simulink model "adaptiverror1 (1)"  (R2025a)
settings: Solver=VariableStepAuto  StartTime=0.0  StopTime=10.0  RelTol=1e-3
undefined symbols (not defined in the file): C1_LUT, C2_LUT, Current_table, OCV_table, R0_LUT, R1_LUT, R2_LUT, SOC_bp, SOC_bp_current, SOC_bp_ocv, Temp_bp
libraries: nesl_utility x13, fl_lib x11, ee_lib x2
settings Model: Creator=nandh  LastModifiedBy=nandh

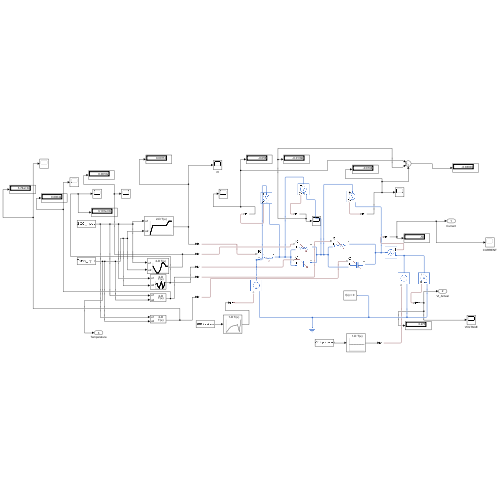
[thumbnail: Simulink's stored preview of the top-level diagram]
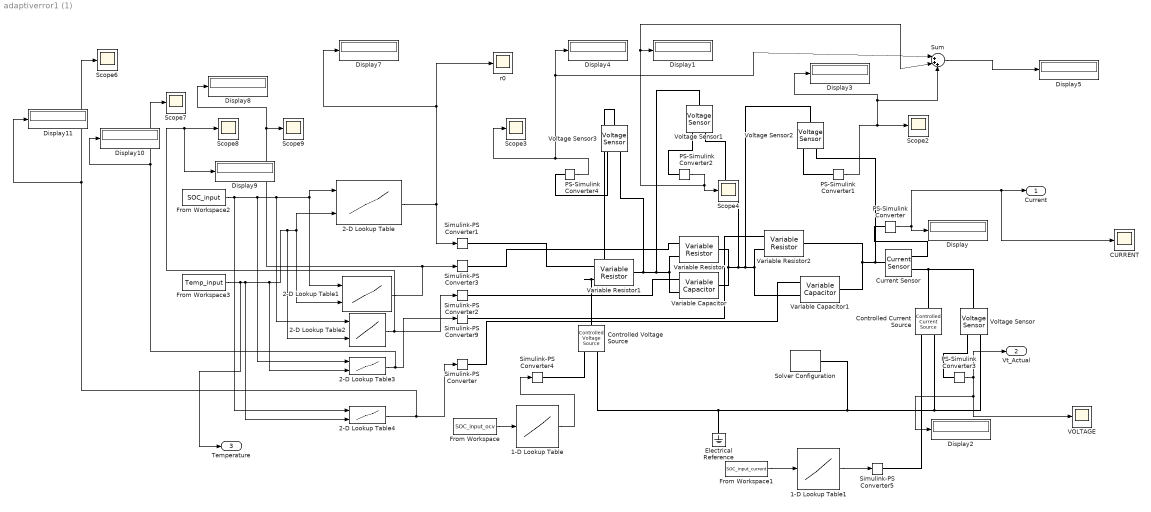
== system adaptiverror1 (1) ==
  1-D Lookup Table : Lookup_n-D  NumberOfTableDimensions=1  BreakpointsForDimension1=SOC_bp_ocv  Table=OCV_table  InternalRulePriority=Speed  RndMeth=Simplest
  1-D Lookup Table1 : Lookup_n-D  NumberOfTableDimensions=1  BreakpointsForDimension1=SOC_bp_current  Table=Current_table  InternalRulePriority=Speed  RndMeth=Simplest
  2-D Lookup Table : Lookup_n-D  BreakpointsForDimension1=SOC_bp  BreakpointsForDimension2=Temp_bp  Table=R0_LUT  InternalRulePriority=Speed  RndMeth=Simplest
      settings: InputPortMap=u0,u1
  2-D Lookup Table1 : Lookup_n-D  BreakpointsForDimension1=SOC_bp  BreakpointsForDimension2=Temp_bp  Table=R1_LUT  InternalRulePriority=Speed  RndMeth=Simplest
      settings: InputPortMap=u0,u1
  2-D Lookup Table2 : Lookup_n-D  BreakpointsForDimension1=SOC_bp  BreakpointsForDimension2=Temp_bp  Table=C1_LUT  InternalRulePriority=Speed  RndMeth=Simplest
      settings: InputPortMap=u0,u1
  2-D Lookup Table3 : Lookup_n-D  BreakpointsForDimension1=SOC_bp  BreakpointsForDimension2=Temp_bp  Table=R2_LUT  InternalRulePriority=Speed  RndMeth=Simplest
      settings: InputPortMap=u0,u1
  2-D Lookup Table4 : Lookup_n-D  BreakpointsForDimension1=SOC_bp  BreakpointsForDimension2=Temp_bp  Table=C2_LUT  InternalRulePriority=Speed  RndMeth=Simplest
      settings: InputPortMap=u0,u1
  CURRENT : Scope
      settings: ActiveDisplayYMinimum=-60  ActiveDisplayYMaximum=-40  DataLoggingVariableName=ScopeData3
  Controlled Current Source : fl_lib/Electrical/Electrical Sources/Controlled Current Source
  Controlled Voltage Source : fl_lib/Electrical/Electrical Sources/Controlled Voltage Source
  Current Sensor : fl_lib/Electrical/Electrical Sensors/Current Sensor
  Display{,1..5,7..11} (11 alike) : Display
  Electrical Reference : fl_lib/Electrical/Electrical Elements/Electrical Reference
  From Workspace : FromWorkspace  VariableName=SOC_input_ocv
  From Workspace1 : FromWorkspace  VariableName=SOC_input_current
  From Workspace2 : FromWorkspace  VariableName=SOC_input  SampleTime=-1
  From Workspace3 : FromWorkspace  VariableName=Temp_input  SampleTime=-1
  PS-Simulink Converter{,1..4} (5 alike) : nesl_utility/PS-Simulink Converter  PhysicalDomain=network_engine_domain  SubClassName=ps_output  LeftPortType=input  RightPortType=output  PseudoPeriodic=off  Frequencies=[]  VectorFormat=inherit  Unit=inherit  AffineConversion=off
  Scope{2..4,6..9} (7 alike) : Scope
      Scope2 settings: DataLoggingVariableName=ScopeData4
      Scope3 settings: ActiveDisplayYMinimum=-1  ActiveDisplayYMaximum=1  DataLoggingVariableName=ScopeData5
      Scope4 settings: ActiveDisplayYMinimum=0.007923423262500005  ActiveDisplayYMaximum=0.1061738716375  DataLoggingVariableName=ScopeData6
      Scope6 settings: ActiveDisplayYMinimum=2871.0870689806384  ActiveDisplayYMaximum=3210.0062898065376  DataLoggingVariableName=ScopeData8
      Scope7 settings: ActiveDisplayYMinimum=0.0024244498599901962  ActiveDisplayYMaximum=0.003217458975094659  DataLoggingVariableName=ScopeData9
      Scope8 settings: ActiveDisplayYMinimum=30443.429999999997  ActiveDisplayYMaximum=31070.130000000005  DataLoggingVariableName=ScopeData10
      Scope9 settings: ActiveDisplayYMinimum=0.00101  ActiveDisplayYMaximum=0.00111  DataLoggingVariableName=ScopeData11
  Simulink-PS Converter{,1..5,9} (7 alike) : nesl_utility/Simulink-PS Converter  PhysicalDomain=network_engine_domain  SubClassName=ps_input  LeftPortType=input  RightPortType=output  PseudoPeriodic=off  Frequencies=[]  NoiseDistribution=none  NoiseParameters=[]  Unit=1  AffineConversion=off  FilteringAndDerivatives=provide  SimscapeFilterOrder=1  InputFilterTimeConstant=0.001  UdotUserProvided=0
  Solver Configuration : nesl_utility/Solver Configuration  PhysicalDomain=network_engine_domain  SubClassName=solver  LeftPortType=input  RightPortType=generic  Tones=[]  Harmonics=[]  SimulateNoise=off  Profile=off  UseLocalSampling=off  EnableSwitchedLinearOptims=on  FrequencyDomain=off  UseCCode=off  RelTol=0.001  AbsTol=0.001  MinStep=1e-09  ToWorkspace=off  RevertToSquareIcSolve=off  NumHomotopyIterations=100  PhasorMode=off  PhasorModeNumHarmonics=1  ConsistencySolver=NEWTON_XTOL_AFTER_FTOL  IndexReductionMethod=DerivativeReplacement  DoDC=off  ResidualTolerance=1e-09  ConsistencyTolSource=GLOBAL  ConsistencyAbsTol=0.001  ConsistencyRelTol=0.001  ConsistencyTolFactor=0.001  UseLocalSolver=off  LocalSolverChoice=NE_BACKWARD_EULER_ADVANCER  ResolveIndetEquations=on  FunctionEvalNumThread=1  LocalSolverSampleTime=0.001  DoFixedCost=off  MaxNonlinIter=3  MaxModeIter=2  ComputeImpulses=off  ImpulseIterations=2  LinearAlgebra=auto  LinearAlgebraNumThread=0  EquationFormulation=NE_TIME_EF  DelaysMemoryBudget=1024  AutomaticFiltering=on  FilteringTimeConstant=0.001  PartitionStorageMethod=AS_NEEDED  PartitionMemoryBudget=1024  PartitionMethod=ROBUST  MultibodyUseLocalSolver=off  MultibodyLocalSolverChoice=ODE1  MultibodyLocalSolverSampleTime=0.001
  Sum : Sum  Inputs=|+++
  VOLTAGE : Scope
      settings: ActiveDisplayYMinimum=3.2573593965369607  ActiveDisplayYMaximum=3.4604043501473822  DataLoggingVariableName=ScopeData2
  Variable Capacitor : ee_lib/Passive/Variable Capacitor  prm=2  Cmin=1e-9 F  r=1e-6 Ohm  v0=0 V  q0=0 C
      settings: InternalSimscapePortConfiguration="{\"Bottom\":[],\"Left\":[{\"id\":\"C\",\"label\":\"C\",\"type\":\"input\"},{\"id\":\"p\",\"label\":\"+\",\"type\":\"foundation.electrical.electrical\"}],\"Right\":[{\"id\":\"n\",\"label\":\"-\",\"type\":\"foundation.electrical.electrical\"}],\"Top\":[]}"
  Variable Capacitor1 : ee_lib/Passive/Variable Capacitor  prm=2  Cmin=1e-9 F  r=1e-6 Ohm  v0=0 V  q0=0 C
      settings: InternalSimscapePortConfiguration="{\"Bottom\":[],\"Left\":[{\"id\":\"C\",\"label\":\"C\",\"type\":\"input\"},{\"id\":\"p\",\"label\":\"+\",\"type\":\"foundation.electrical.electrical\"}],\"Right\":[{\"id\":\"n\",\"label\":\"-\",\"type\":\"foundation.electrical.electrical\"}],\"Top\":[]}"
  Variable Resistor : fl_lib/Electrical/Electrical Elements/Variable Resistor  Rmin=0 Ohm  thermalEnable=false  thermal_mass=1 J/K  i_specify=off  i_priority=None  i=0 A  i_nominal_specify=off  i_nominal_value=1  i_nominal_unit=A  v_specify=off  v_priority=None  v=0 V  v_nominal_specify=off  v_nominal_value=1  v_nominal_unit=V  T_specify=off  T_priority=None  T=300 K  T_nominal_specify=off  T_nominal_value=1  T_nominal_unit=K
  Variable Resistor1 : fl_lib/Electrical/Electrical Elements/Variable Resistor  Rmin=0 Ohm  thermalEnable=false  thermal_mass=1 J/K  i_specify=off  i_priority=None  i=0 A  i_nominal_specify=off  i_nominal_value=1  i_nominal_unit=A  v_specify=off  v_priority=None  v=0 V  v_nominal_specify=off  v_nominal_value=1  v_nominal_unit=V  T_specify=off  T_priority=None  T=300 K  T_nominal_specify=off  T_nominal_value=1  T_nominal_unit=K
  Variable Resistor2 : fl_lib/Electrical/Electrical Elements/Variable Resistor  Rmin=0 Ohm  thermalEnable=false  thermal_mass=1 J/K  i_specify=off  i_priority=None  i=0 A  i_nominal_specify=off  i_nominal_value=1  i_nominal_unit=A  v_specify=off  v_priority=None  v=0 V  v_nominal_specify=off  v_nominal_value=1  v_nominal_unit=V  T_specify=off  T_priority=None  T=300 K  T_nominal_specify=off  T_nominal_value=1  T_nominal_unit=K
  Voltage Sensor{,1..3} (4 alike) : fl_lib/Electrical/Electrical Sensors/Voltage Sensor
  r0 : Scope
      settings: ActiveDisplayYMinimum=0.0063433679673202247  ActiveDisplayYMaximum=0.007013413404943894  DataLoggingVariableName=ScopeData7
  Current : Outport
  Vt_Actual : Outport  Port=2
  Temperature : Outport  Port=3
  wires:
  PS-Simulink Converter1/1 -> Sum/3, Display3/1, Scope2/1
  2-D Lookup Table/1 -> Simulink-PS Converter1/1, Display7/1, r0/1
  From Workspace2/1 -> 2-D Lookup Table4/1, 2-D Lookup Table3/1, 2-D Lookup Table2/1, 2-D Lookup Table1/1, 2-D Lookup Table/1
  2-D Lookup Table1/1 -> Simulink-PS Converter3/1, Display8/1, Scope9/1
  2-D Lookup Table4/1 -> Display11/1, Scope6/1, Simulink-PS Converter/1
  2-D Lookup Table3/1 -> Display10/1, Scope7/1, Simulink-PS Converter9/1
  From Workspace3/1 -> Temperature/1, 2-D Lookup Table4/2, 2-D Lookup Table3/2, 2-D Lookup Table/2, 2-D Lookup Table1/2, 2-D Lookup Table2/2
  Sum/1 -> Display5/1
  2-D Lookup Table2/1 -> Display9/1, Scope8/1, Simulink-PS Converter2/1
  PS-Simulink Converter2/1 -> Sum/2, Display1/1, Scope4/1
  PS-Simulink Converter4/1 -> Sum/1, Display4/1, Scope3/1
  PS-Simulink Converter/1 -> CURRENT/1, Current/1, Display/1
  PS-Simulink Converter3/1 -> Vt_Actual/1, VOLTAGE/1, Display2/1
  From Workspace/1 -> 1-D Lookup Table/1
  1-D Lookup Table/1 -> Simulink-PS Converter4/1
  From Workspace1/1 -> 1-D Lookup Table1/1
  1-D Lookup Table1/1 -> Simulink-PS Converter5/1
  connections:
  Variable Resistor2/RConn1 -- Current Sensor/LConn1 -- Voltage Sensor2/RConn2 -- Variable Capacitor1/RConn1
  Variable Resistor1/LConn2 -- Controlled Voltage Source/LConn1 -- Voltage Sensor3/LConn1
  Variable Resistor1/RConn1 -- Variable Capacitor/LConn2 -- Variable Resistor/LConn2 -- Voltage Sensor1/LConn1 -- Voltage Sensor3/RConn2
  Voltage Sensor1/RConn2 -- Variable Resistor/RConn1 -- Variable Capacitor/RConn1 -- Voltage Sensor2/LConn1 -- Variable Resistor2/LConn2 -- Variable Capacitor1/LConn2
  Voltage Sensor/LConn1 -- Current Sensor/RConn2 -- Controlled Current Source/LConn1
  Voltage Sensor/RConn2 -- Electrical Reference/LConn1 -- Controlled Voltage Source/RConn2 -- Solver Configuration/RConn1 -- Controlled Current Source/RConn2
  Simulink-PS Converter1/RConn1 -- Variable Resistor1/LConn1
  Simulink-PS Converter3/RConn1 -- Variable Resistor/LConn1
  Voltage Sensor3/RConn1 -- PS-Simulink Converter4/LConn1
  Voltage Sensor/RConn1 -- PS-Simulink Converter3/LConn1
  Simulink-PS Converter9/RConn1 -- Variable Resistor2/LConn1
  Voltage Sensor1/RConn1 -- PS-Simulink Converter2/LConn1
  Simulink-PS Converter/RConn1 -- Variable Capacitor1/LConn1
  Simulink-PS Converter2/RConn1 -- Variable Capacitor/LConn1
  Voltage Sensor2/RConn1 -- PS-Simulink Converter1/LConn1
  Simulink-PS Converter4/RConn1 -- Controlled Voltage Source/RConn1
  Current Sensor/RConn1 -- PS-Simulink Converter/LConn1
  Simulink-PS Converter5/RConn1 -- Controlled Current Source/RConn1
